simulink model "rsbq2"  (R2021a)
settings: Solver=FixedStepDiscrete  StartTime=0.0  StopTime=7.5  RelTol=1e-3  EnableMultiTasking=on
undefined symbols (not defined in the file): b
libraries: commsrccod2 x2, simulink_extras x1, dsparch4 x1
settings Model: Creator=sebastienroy  LastModifiedBy=roys2121
settings SolverCC: AlgebraicLoopSolver=TrustRegion
settings DataIOCC: LimitDataPoints=on  SaveFormat=Array  ReturnWorkspaceOutputs=off
settings OptimizationCC: LifeSpan=inf
settings DebuggingCC: UnderspecifiedInitializationDetection=Classic  MergeDetectMultiDrivingBlocksExec=none  SolverPrmCheckMsg=warning  StateNameClashWarn=warning  SFUnexpectedBacktrackingDiag=warning  SFNoUnconditionalDefaultTransitionDiag=warning  SFExecutionAtInitializationDiag=none  SFMachineParentedDataDiag=warning  ArithmeticOperatorsInVariantConditions=warning
settings HardwareCC: ProdBitPerPointer=32  ProdBitPerSizeT=32  ProdBitPerPtrDiffT=32  ProdLargestAtomicFloat=None  ProdIntDivRoundTo=Undefined  ProdEndianess=Unspecified  ProdWordSize=32  ProdHWDeviceType=32-bit Generic
settings ModelReferenceCC: PropagateSignalLabelsOutOfModel=off
settings SFSimCC: SimUseLocalCustomCode=off  CustomCodeUndefinedFunction=UseInterfaceOnly
settings RTWCC: RTWUseLocalCustomCode=off
settings CodeAppCC: StateflowObjectComments=on
settings GRTTargetCC: TargetLangStandard=C89/C90 (ANSI)
settings ConfigComp: CovMetricSettings=dw  CovSaveCumulativeToWorkspaceVar=on  CovSaveSingleToWorkspaceVar=on  CovExternalEMLEnable=off

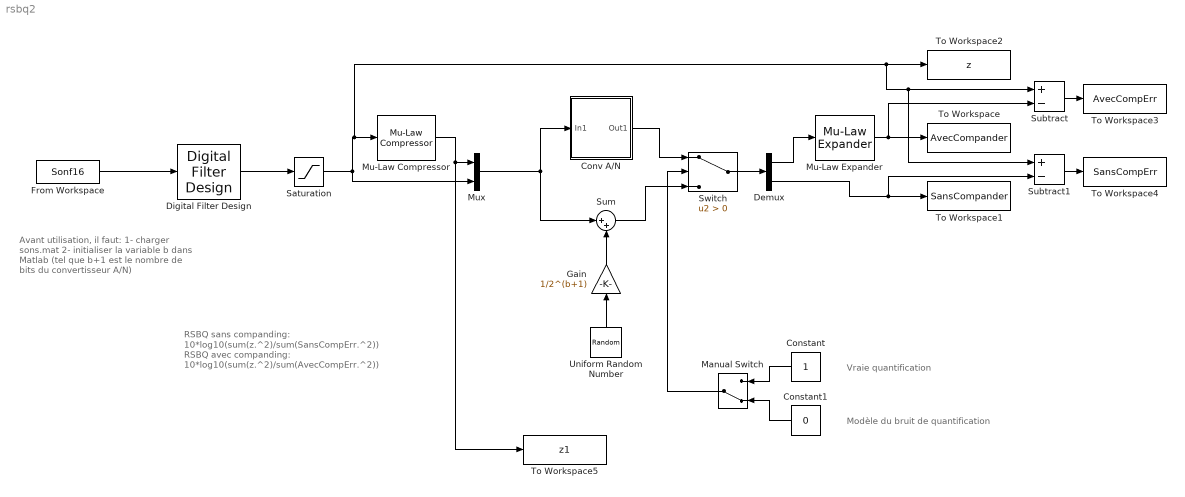
== system rsbq2 ==
  note: Avant utilisation, il faut:
      | 1- charger sons.mat
      | 2- initialiser la variable b dans Matlab
      | (tel que b+1 est le nombre de bits du
      | convertisseur A/N)
  note: Modèle du bruit de quantification
  note: Vraie quantification
  note: RSBQ sans companding:
      |
      | 10*log10(sum(z.^2)/sum(SansCompErr.^2))
      |
      | RSBQ avec companding:
      |
      | 10*log10(sum(z.^2)/sum(AvecCompErr.^2))
  Constant : Constant
  Constant1 : Constant  Value=0
  Conv A/N : Subsystem
  Demux : Demux  Outputs=2
  Digital Filter Design : dsparch4/Digital Filter Design  mwdsp_browser_bugfix_var=off
  From Workspace : FromWorkspace  VariableName=Sonf16  SampleTime=6.25e-5  Interpolate=off  OutputAfterFinalValue=Setting to zero
  Gain : Gain  Gain=1/2^(b+1)
  Manual Switch : ManualSwitch  CurrentSetting=0
  Mu-Law Compressor : commsrccod2/Mu-Law Compressor  mu=255  V=1
      settings: SourceProductBaseCode=CM
  Mu-Law Expander : commsrccod2/Mu-Law Expander  mu=255  V=1
      settings: SourceProductBaseCode=CM
  Mux : Mux  Inputs=2
  Saturation : Saturate  UpperLimit=1  LowerLimit=-1
  Subtract : Sum  Inputs=+-
  Subtract1 : Sum  Inputs=+-
  Sum : Sum  Inputs=|++
  Switch : Switch  Criteria=u2 > Threshold
  To Workspace : ToWorkspace  VariableName=AvecCompander  SampleTime=-1
      settings: Save2DSignal=2-D array (concatenate along first dimension)
  To Workspace1 : ToWorkspace  VariableName=SansCompander  SampleTime=-1
  To Workspace2 : ToWorkspace  VariableName=z  SampleTime=-1
  To Workspace3 : ToWorkspace  VariableName=AvecCompErr  SampleTime=-1
      settings: Save2DSignal=2-D array (concatenate along first dimension)
  To Workspace4 : ToWorkspace  VariableName=SansCompErr  SampleTime=-1
      settings: Save2DSignal=2-D array (concatenate along first dimension)
  To Workspace5 : ToWorkspace  VariableName=z1  SampleTime=-1
  Uniform Random Number : UniformRandomNumber  SampleTime=6.25e-5
  wires:
  Mu-Law Compressor/1 -> To Workspace5/1, Mux/1
  From Workspace/1 -> Digital Filter Design/1
  Demux/1 -> Mu-Law Expander/1
  Mu-Law Expander/1 -> Subtract/2, To Workspace/1
  Demux/2 -> Subtract1/2, To Workspace1/1
  Subtract/1 -> To Workspace3/1
  Subtract1/1 -> To Workspace4/1
  Switch/1 -> Demux/1
  Conv A/N/1(Out1) -> Switch/1
  Mux/1 -> Sum/1, Conv A/N/1(In1)
  Uniform Random Number/1 -> Gain/1
  Gain/1 -> Sum/2
  Saturation/1 -> Subtract1/1, Subtract/1, To Workspace2/1, Mu-Law Compressor/1, Mux/2
  Digital Filter Design/1 -> Saturation/1
  Sum/1 -> Switch/3
  Manual Switch/1 -> Switch/2
  Constant/1 -> Manual Switch/1
  Constant1/1 -> Manual Switch/2

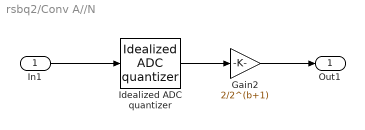
== system rsbq2/Conv A//N ==
  In1 : Inport
  Gain2 : Gain  Gain=2/2^(b+1)
  Idealized ADC quantizer : simulink_extras/Additional Discrete/Idealized ADC quantizer  NumberOfConverterBits=b+1  Vmin=-1  Vmax=1  OutputDataType=double  OutputNegativeValues=on
  Out1 : Outport  VectorParamsAs1DForOutWhenUnconnected=off
  wires:
  Idealized ADC quantizer/1 -> Gain2/1
  Gain2/1 -> Out1/1
  In1/1 -> Idealized ADC quantizer/1
